simulink subsystem "ForwardDynamics"  (R2022a)
settings: Solver=VariableStepAuto  StartTime=0.0  StopTime=10.0  RelTol=1e-3
model mask{spaceRobot=SpaceRobot, SimulateUsing=Code generation}
  mask prompts: SimulateUsing "SystemBlock:MATLABSystem:SimulateUsing"
settings Model: Creator=charl  LastModifiedBy=charl

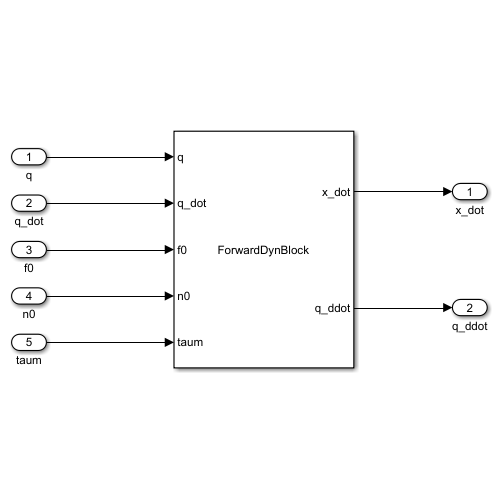
[thumbnail: Simulink's stored preview of the top-level diagram]
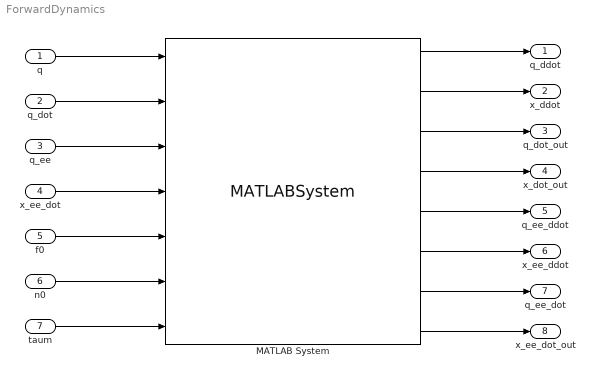
== system ForwardDynamics ==
  q : Inport
  q_dot : Inport  Port=2
  q_ee : Inport  Port=3
  x_ee_dot : Inport  Port=4
  f0 : Inport  Port=5
  n0 : Inport  Port=6
  taum : Inport  Port=7
  MATLAB System : MATLABSystem  System=ForwardDynBlock  srInfo=srInfo  srInfoFunc=srInfoFunc  srStateFunc=srStateFunc  srStateFuncMex=srStateFuncMex  SimulateUsing=Interpreted execution
      mask Type: ForwardDynBlock
      mask Display:
      | disp('ForwardDynBlock');
      | port_label('input',1,'q');
      | port_label('input',2,'q_dot');
      | port_label('input',3,'q_ee');
      | port_label('input',4,'x_ee_dot');
      | port_label('input',5,'f0');
      | port_label('input',6,'n0');
      | port_label('input',7,'taum');
      | port_label('output',1,'q_ddot');
      | port_label('output',2,'x_ddot');
      | port_label('output',3,'q_dot');
      | port_label('output',4,'x_dot');
      | port_label('output',5,'q_ee_ddot');
      | port_label('output',6,'x_ee_ddot');
      | port_label('output',7,'q_ee_dot');
      | port_label('output',8,'x_ee_dot');
  q_ddot : Outport
  x_ddot : Outport  Port=2
  q_dot_out : Outport  Port=3
  x_dot_out : Outport  Port=4
  q_ee_ddot : Outport  Port=5
  x_ee_ddot : Outport  Port=6
  q_ee_dot : Outport  Port=7
  x_ee_dot_out : Outport  Port=8
  wires:
  MATLAB System/8 -> x_ee_dot_out/1
  MATLAB System/7 -> q_ee_dot/1
  MATLAB System/6 -> x_ee_ddot/1
  MATLAB System/5 -> q_ee_ddot/1
  MATLAB System/4 -> x_dot_out/1
  MATLAB System/2 -> x_ddot/1
  MATLAB System/3 -> q_dot_out/1
  taum/1 -> MATLAB System/7
  n0/1 -> MATLAB System/6
  x_ee_dot/1 -> MATLAB System/4
  q_ee/1 -> MATLAB System/3
  MATLAB System/1 -> q_ddot/1
  q_dot/1 -> MATLAB System/2
  q/1 -> MATLAB System/1
  f0/1 -> MATLAB System/5
